simulink model "Battery_Model"  (R2023b)
settings: Solver=VariableStepAuto  StartTime=0.0  StopTime=10.0  RelTol=1e-3
values from neighbouring files (symbols this model uses):
  Capacity = 5    [Battery_Mod.m]
  R_bat = 0.5    [Battery_Mod.m]
  V_in = 12    [Battery_Mod.m]
settings Model: Creator=mdhel  LastModifiedBy=mdhel

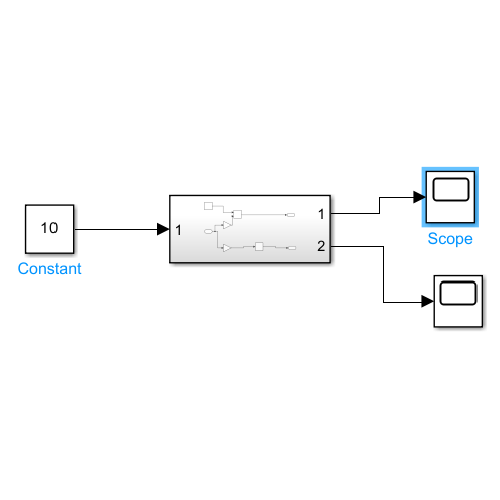
[thumbnail: Simulink's stored preview of the top-level diagram]
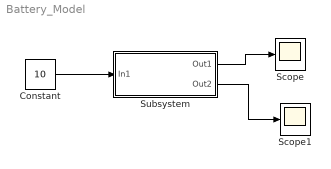
== system Battery_Model ==
  Constant : Constant  Value=10
  Scope : Scope
  Scope1 : Scope
  Subsystem : Subsystem
  wires:
  Constant/1 -> Subsystem/1(In1)
  Subsystem/1(Out1) -> Scope/1
  Subsystem/2(Out2) -> Scope1/1

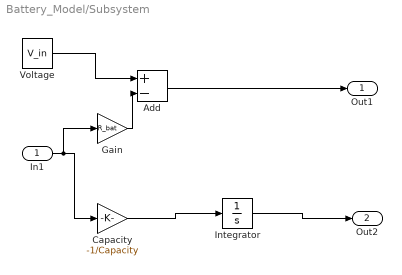
== system Battery_Model/Subsystem ==
  In1 : Inport
  Add : Sum  Inputs=+-
  Capacity : Gain  Gain=-1/Capacity
  Gain : Gain  Gain=R_bat
  Integrator : Integrator  InitialCondition=1
  Voltage : Constant  Value=V_in
  Out1 : Outport
  Out2 : Outport  Port=2
  wires:
  Voltage/1 -> Add/1
  Add/1 -> Out1/1
  Capacity/1 -> Integrator/1
  Integrator/1 -> Out2/1
  In1/1 -> Gain/1, Capacity/1
  Gain/1 -> Add/2
